simulink model "MSBR"  (R2015b)
settings: Solver=ode45  StartTime=0.0  StopTime=simtime  RelTol=1e-3
values from neighbouring files (symbols this model uses):
  a_b = 1.656E-05    (= 1.656e-05)    [Parameters_Core_PHE.m]    (also in Parameters_Core_PHE_FEHE.m; Parameters_MSBR.m)
  a_f = -8.172E-05    (= -8.172e-05)    [Parameters_Core_PHE.m]    (also in Parameters_Core_PHE_FEHE.m; Parameters_MSBR.m)
  a_g = 2.016E-05    (= 2.016e-05)    [Parameters_Core_PHE.m]    (also in Parameters_Core_PHE_FEHE.m; Parameters_MSBR.m)
  beta = [2.290E-04, 8.320E-04, 7.100E-04, 8.520E-04, 1.710E-04, 1.020E-04]    [Parameters_Core_PHE.m]    (also in Parameters_Core_PHE_FEHE.m; Parameters_MSBR.m)
  beta_t = sum(beta)    [Parameters_Core_PHE.m]    (also in Parameters_Core_PHE_FEHE.m; Parameters_MSBR.m)
  hA_bg = 1.054E+00    (= 1.054)    [Parameters_Core_PHE.m]    (also in Parameters_Core_PHE_FEHE.m; Parameters_MSBR.m)
  hA_fg_dn = 1.123E+00    (= 1.123)    [Parameters_Core_PHE.m]    (also in Parameters_Core_PHE_FEHE.m; Parameters_MSBR.m)
  hA_fg_up = 1.733E+00    (= 1.733)    [Parameters_Core_PHE.m]    (also in Parameters_Core_PHE_FEHE.m; Parameters_MSBR.m)
  hA_p1 = 0.75*3.030    (= 2.2725)    [Parameters_Core_PHE.m]    (also in Parameters_Core_PHE_FEHE.m = 2.993352; Parameters_MSBR.m = 2.993352; Parameters_PHE.m = 3.03)
  hA_p2 = 0.75*3.030    (= 2.2725)    [Parameters_Core_PHE.m]    (also in Parameters_Core_PHE_FEHE.m = 2.993352; Parameters_MSBR.m = 2.993352; Parameters_PHE.m = 3.03)
  hA_p3 = 0.75*3.030    (= 2.2725)    [Parameters_Core_PHE.m]    (also in Parameters_Core_PHE_FEHE.m = 2.993352; Parameters_MSBR.m = 2.993352; Parameters_PHE.m = 3.03)
  hA_p4 = 0.75*3.030    (= 2.2725)    [Parameters_Core_PHE.m]    (also in Parameters_Core_PHE_FEHE.m = 2.993352; Parameters_MSBR.m = 2.993352; Parameters_PHE.m = 3.03)
  hA_pb1 = 7.150E-01    (= 0.715)    [Parameters_Core_PHE_FEHE.m]    (also in Parameters_MSBR.m)
  hA_pb2 = 7.150E-01    (= 0.715)    [Parameters_Core_PHE_FEHE.m]    (also in Parameters_MSBR.m)
  hA_s1 = 0.75*5.929    (= 4.44675)    [Parameters_Core_PHE.m]    (also in Parameters_Core_PHE_FEHE.m = 5.85606; Parameters_MSBR.m = 5.85606; Parameters_PHE.m = 5.929)
  hA_s2 = 0.75*5.929    (= 4.44675)    [Parameters_Core_PHE.m]    (also in Parameters_Core_PHE_FEHE.m = 5.85606; Parameters_MSBR.m = 5.85606; Parameters_PHE.m = 5.929)
  hA_s3 = 0.75*5.929    (= 4.44675)    [Parameters_Core_PHE.m]    (also in Parameters_Core_PHE_FEHE.m = 5.85606; Parameters_MSBR.m = 5.85606; Parameters_PHE.m = 5.929)
  hA_s4 = 0.75*5.929    (= 4.44675)    [Parameters_Core_PHE.m]    (also in Parameters_Core_PHE_FEHE.m = 5.85606; Parameters_MSBR.m = 5.85606; Parameters_PHE.m = 5.929)
  hA_s5 = 7.150E-01    (= 0.715)    [Parameters_Core_PHE_FEHE.m]    (also in Parameters_MSBR.m)
  hA_s6 = 7.150E-01    (= 0.715)    [Parameters_Core_PHE_FEHE.m]    (also in Parameters_MSBR.m)
  k_1 = 5.000E-01    (= 0.5)    [Parameters_Core_PHE.m]    (also in Parameters_Core_PHE_FEHE.m; Parameters_MSBR.m)
  k_1b = 5.000E-01    (= 0.5)    [Parameters_Core_PHE.m]    (also in Parameters_Core_PHE_FEHE.m; Parameters_MSBR.m)
  k_2 = 5.000E-01    (= 0.5)    [Parameters_Core_PHE.m]    (also in Parameters_Core_PHE_FEHE.m; Parameters_MSBR.m)
  k_2b = 5.000E-01    (= 0.5)    [Parameters_Core_PHE.m]    (also in Parameters_Core_PHE_FEHE.m; Parameters_MSBR.m)
  k_3 = 5.000E-01    (= 0.5)    [Parameters_Core_PHE.m]    (also in Parameters_Core_PHE_FEHE.m; Parameters_MSBR.m)
  k_4 = 5.000E-01    (= 0.5)    [Parameters_Core_PHE.m]    (also in Parameters_Core_PHE_FEHE.m; Parameters_MSBR.m)
  k_b1 = 8.500E-03    (= 0.0085)    [Parameters_Core_PHE.m]    (also in Parameters_Core_PHE_FEHE.m; Parameters_MSBR.m)
  k_b2 = 8.500E-03    (= 0.0085)    [Parameters_Core_PHE.m]    (also in Parameters_Core_PHE_FEHE.m; Parameters_MSBR.m)
  k_f1 = 2.210E-01    (= 0.221)    [Parameters_Core_PHE.m]    (also in Parameters_Core_PHE_FEHE.m; Parameters_MSBR.m)
  k_f2 = 2.210E-01    (= 0.221)    [Parameters_Core_PHE.m]    (also in Parameters_Core_PHE_FEHE.m; Parameters_MSBR.m)
  k_f3 = 2.210E-01    (= 0.221)    [Parameters_Core_PHE.m]    (also in Parameters_Core_PHE_FEHE.m; Parameters_MSBR.m)
  k_f4 = 2.210E-01    (= 0.221)    [Parameters_Core_PHE.m]    (also in Parameters_Core_PHE_FEHE.m; Parameters_MSBR.m)
  k_g1 = 3.300E-02    (= 0.033)    [Parameters_Core_PHE.m]    (also in Parameters_Core_PHE_FEHE.m; Parameters_MSBR.m)
  k_g2 = 3.300E-02    (= 0.033)    [Parameters_Core_PHE.m]    (also in Parameters_Core_PHE_FEHE.m; Parameters_MSBR.m)
  k_g3 = 8.140E-03    (= 0.00814)    [Parameters_Core_PHE.m]    (also in Parameters_Core_PHE_FEHE.m; Parameters_MSBR.m)
  Lam = 3.300E-04    (= 0.00033)    [Parameters_Core_PHE.m]    (also in Parameters_Core_PHE_FEHE.m; Parameters_MSBR.m)
  lam = [1.260E-02, 3.370E-02, 1.390E-01, 3.250E-01, 1.130E+00, 2.500E+00]    [Parameters_Core_PHE.m]    (also in Parameters_Core_PHE_FEHE.m; Parameters_MSBR.m)
  mb_cpb = 3.297E+01    (= 32.97)    [Parameters_Core_PHE_FEHE.m]    (also in Parameters_MSBR.m)
  mcp_b1 = 1.733E+00    (= 1.733)    [Parameters_Core_PHE.m]    (also in Parameters_Core_PHE_FEHE.m; Parameters_MSBR.m)
  mcp_b2 = 1.733E+00    (= 1.733)    [Parameters_Core_PHE.m]    (also in Parameters_Core_PHE_FEHE.m; Parameters_MSBR.m)
  mcp_f1 = 2.748E-01    (= 0.2748)    [Parameters_Core_PHE.m]    (also in Parameters_Core_PHE_FEHE.m; Parameters_MSBR.m)
  mcp_f2 = 2.748E-01    (= 0.2748)    [Parameters_Core_PHE.m]    (also in Parameters_Core_PHE_FEHE.m; Parameters_MSBR.m)
  mcp_f3 = 2.748E-01    (= 0.2748)    [Parameters_Core_PHE.m]    (also in Parameters_Core_PHE_FEHE.m; Parameters_MSBR.m)
  mcp_f4 = 2.748E-01    (= 0.2748)    [Parameters_Core_PHE.m]    (also in Parameters_Core_PHE_FEHE.m; Parameters_MSBR.m)
  mcp_g1 = 1.403E+01    (= 14.03)    [Parameters_Core_PHE.m]    (also in Parameters_Core_PHE_FEHE.m; Parameters_MSBR.m)
  mcp_g2 = 1.403E+01    (= 14.03)    [Parameters_Core_PHE.m]    (also in Parameters_Core_PHE_FEHE.m; Parameters_MSBR.m)
  mcp_g3 = 3.467E+00    (= 3.467)    [Parameters_Core_PHE.m]    (also in Parameters_Core_PHE_FEHE.m; Parameters_MSBR.m)
  mcp_p1 = mn_p*cp_p    (= 1.743765)    [Parameters_Core_PHE.m]    (also in Parameters_Core_PHE_FEHE.m; Parameters_MSBR.m; Parameters_PHE.m = 0.930008)
  mcp_p2 = mn_p*cp_p    (= 1.743765)    [Parameters_Core_PHE.m]    (also in Parameters_Core_PHE_FEHE.m; Parameters_MSBR.m; Parameters_PHE.m = 0.930008)
  mcp_p3 = mn_p*cp_p    (= 1.743765)    [Parameters_Core_PHE.m]    (also in Parameters_Core_PHE_FEHE.m; Parameters_MSBR.m; Parameters_PHE.m = 0.930008)
  mcp_p4 = mn_p*cp_p    (= 1.743765)    [Parameters_Core_PHE.m]    (also in Parameters_Core_PHE_FEHE.m; Parameters_MSBR.m; Parameters_PHE.m = 0.930008)
  mcp_pb1 = 3.967E-01    (= 0.3967)    [Parameters_Core_PHE_FEHE.m]    (also in Parameters_MSBR.m)
  mcp_pb2 = 3.967E-01    (= 0.3967)    [Parameters_Core_PHE_FEHE.m]    (also in Parameters_MSBR.m)
  mcp_s1 = mn_s*cp_s    (= 6.80458)    [Parameters_Core_PHE.m]    (also in Parameters_Core_PHE_FEHE.m; Parameters_MSBR.m; Parameters_PHE.m)
  mcp_s2 = mn_s*cp_s    (= 6.80458)    [Parameters_Core_PHE.m]    (also in Parameters_Core_PHE_FEHE.m; Parameters_MSBR.m; Parameters_PHE.m)
  mcp_s3 = mn_s*cp_s    (= 6.80458)    [Parameters_Core_PHE.m]    (also in Parameters_Core_PHE_FEHE.m; Parameters_MSBR.m; Parameters_PHE.m)
  mcp_s4 = mn_s*cp_s    (= 6.80458)    [Parameters_Core_PHE.m]    (also in Parameters_Core_PHE_FEHE.m; Parameters_MSBR.m; Parameters_PHE.m)
  mcp_s5 = 2.632E+00    (= 2.632)    [Parameters_Core_PHE_FEHE.m]    (also in Parameters_MSBR.m)
  mcp_s6 = 2.632E+00    (= 2.632)    [Parameters_Core_PHE_FEHE.m]    (also in Parameters_MSBR.m)
  mcp_t1 = 2.158    [Parameters_Core_PHE.m]    (also in Parameters_Core_PHE_FEHE.m; Parameters_MSBR.m; Parameters_PHE.m)
  mcp_t2 = 2.158    [Parameters_Core_PHE.m]    (also in Parameters_Core_PHE_FEHE.m; Parameters_MSBR.m; Parameters_PHE.m)
  mcp_t3 = m_t*cp_t    (= 0.51412242)    [Parameters_Core_PHE_FEHE.m]    (also in Parameters_MSBR.m)
  mn_m = 1.414e3    (= 1414)    [Parameters_Core_PHE.m]    (also in Parameters_Core_PHE_FEHE.m; Parameters_MSBR.m; Parameters_PHE.m)
  mn_ms = mn_m    (= 1414)    [Parameters_Core_PHE_FEHE.m]    (also in Parameters_MSBR.m)
  mn_p = m_p/nn_p    (= 757.5)    [Parameters_Core_PHE.m]    (also in Parameters_Core_PHE_FEHE.m; Parameters_MSBR.m; Parameters_PHE.m = 404)
  mn_s = m_s/nn_s    (= 3970)    [Parameters_Core_PHE.m]    (also in Parameters_Core_PHE_FEHE.m; Parameters_MSBR.m; Parameters_PHE.m)
  mr_cpr = 1.050E+01    (= 10.5)    [Parameters_Core_PHE_FEHE.m]    (also in Parameters_MSBR.m)
  n_frac0 = 1    [Parameters_Core_PHE.m]    (also in Parameters_Core_PHE_FEHE.m; Parameters_MSBR.m)
  P = 556.0    (= 556)    [Parameters_Core_PHE.m]    (also in Parameters_Core_PHE_FEHE.m; Parameters_MSBR.m)
  p_b = 0.87*P    (= 483.72)    [Parameters_Core_PHE_FEHE.m]    (also in Parameters_MSBR.m)
  p_r = 0.13*P    (= 72.28)    [Parameters_Core_PHE_FEHE.m]    (also in Parameters_MSBR.m)
  T0_b1 = 648.88    [Parameters_Core_PHE.m]    (also in Parameters_Core_PHE_FEHE.m; Parameters_MSBR.m)
  T0_b2 = 676.66    [Parameters_Core_PHE.m]    (also in Parameters_Core_PHE_FEHE.m; Parameters_MSBR.m)
  T0_f1 = 579.44    [Parameters_Core_PHE.m]    (also in Parameters_Core_PHE_FEHE.m; Parameters_MSBR.m)
  T0_f2 = 621.11    [Parameters_Core_PHE.m]    (also in Parameters_Core_PHE_FEHE.m; Parameters_MSBR.m)
  T0_f3 = 662.77    [Parameters_Core_PHE.m]    (also in Parameters_Core_PHE_FEHE.m; Parameters_MSBR.m)
  T0_f4 = 704.44    [Parameters_Core_PHE.m]    (also in Parameters_Core_PHE_FEHE.m; Parameters_MSBR.m)
  T0_g1 = 590.00    (= 590)    [Parameters_Core_PHE.m]    (also in Parameters_Core_PHE_FEHE.m; Parameters_MSBR.m)
  T0_g2 = 673.33    [Parameters_Core_PHE.m]    (also in Parameters_Core_PHE_FEHE.m; Parameters_MSBR.m)
  T0_g3 = 652.77    [Parameters_Core_PHE.m]    (also in Parameters_Core_PHE_FEHE.m; Parameters_MSBR.m)
  T0_p1 = Tp_in - 41.6675    (= 662.7725)    [Parameters_Core_PHE.m]    (also in Parameters_Core_PHE_FEHE.m; Parameters_MSBR.m; Parameters_PHE.m)
  T0_p2 = Tp_in - 2*41.6675    (= 621.105)    [Parameters_Core_PHE.m]    (also in Parameters_Core_PHE_FEHE.m; Parameters_MSBR.m; Parameters_PHE.m)
  T0_p3 = Tp_in - 3*41.6675    (= 579.4375)    [Parameters_Core_PHE.m]    (also in Parameters_Core_PHE_FEHE.m; Parameters_MSBR.m; Parameters_PHE.m)
  T0_p4 = 537.77    [Parameters_Core_PHE.m]    (also in Parameters_Core_PHE_FEHE.m; Parameters_MSBR.m; Parameters_PHE.m)
  T0_pb1 = 648.88    [Parameters_Core_PHE_FEHE.m]    (also in Parameters_MSBR.m)
  T0_pb2 = 676.66    [Parameters_Core_PHE_FEHE.m]    (also in Parameters_MSBR.m)
  T0_pm = T0_p2    (= 621.105)    [Parameters_Core_PHE.m]    (also in Parameters_Core_PHE_FEHE.m; Parameters_MSBR.m; Parameters_PHE.m)
  T0_s1 = Ts_in + 36.25    (= 490.694)    [Parameters_Core_PHE.m]    (also in Parameters_Core_PHE_FEHE.m; Parameters_MSBR.m; Parameters_PHE.m)
  T0_s2 = Ts_in + 2*36.25    (= 526.944)    [Parameters_Core_PHE.m]    (also in Parameters_Core_PHE_FEHE.m; Parameters_MSBR.m; Parameters_PHE.m)
  T0_s3 = Ts_in + 3*36.25    (= 563.194)    [Parameters_Core_PHE.m]    (also in Parameters_Core_PHE_FEHE.m; Parameters_MSBR.m; Parameters_PHE.m)
  T0_s4 = 599.4444    [Parameters_Core_PHE.m]    (also in Parameters_Core_PHE_FEHE.m; Parameters_MSBR.m; Parameters_PHE.m)
  T0_s5 = 603.33    [Parameters_Core_PHE_FEHE.m]    (also in Parameters_MSBR.m)
  T0_s6 = 607.22    [Parameters_Core_PHE_FEHE.m]    (also in Parameters_MSBR.m)
  T0_t1 = 596.87    [Parameters_Core_PHE.m]    (also in Parameters_Core_PHE_FEHE.m; Parameters_MSBR.m; Parameters_PHE.m)
  T0_t2 = 520.71    [Parameters_Core_PHE.m]    (also in Parameters_Core_PHE_FEHE.m; Parameters_MSBR.m; Parameters_PHE.m)
  T0_t3 = 633.6967    [Parameters_Core_PHE_FEHE.m]    (also in Parameters_MSBR.m)
  tau_1 = mn_f/W_f    (= 0.084441301273)    [Parameters_Core_PHE.m]    (also in Parameters_Core_PHE_FEHE.m; Parameters_MSBR.m)
  tau_2 = mn_f/W_f    (= 0.084441301273)    [Parameters_Core_PHE.m]    (also in Parameters_Core_PHE_FEHE.m; Parameters_MSBR.m)
  tau_3 = mn_f/W_f    (= 0.084441301273)    [Parameters_Core_PHE.m]    (also in Parameters_Core_PHE_FEHE.m; Parameters_MSBR.m)
  tau_4 = mn_f/W_f    (= 0.084441301273)    [Parameters_Core_PHE.m]    (also in Parameters_Core_PHE_FEHE.m; Parameters_MSBR.m)
  tau_b = 10.43    [Parameters_Core_PHE_FEHE.m]    (also in Parameters_MSBR.m)
  tau_b1 = 6.998E+00    (= 6.998)    [Parameters_Core_PHE.m]    (also in Parameters_Core_PHE_FEHE.m; Parameters_MSBR.m)
  tau_b2 = 6.998E+00    (= 6.998)    [Parameters_Core_PHE.m]    (also in Parameters_Core_PHE_FEHE.m; Parameters_MSBR.m)
  tau_b_fhx = 4.2    [Parameters_Core_PHE.m]    (also in Parameters_Core_PHE_FEHE.m; Parameters_MSBR.m)
  tau_c = 3.28    [Parameters_Core_PHE.m]    (also in Parameters_Core_PHE_FEHE.m; Parameters_MSBR.m)
  tau_c_fehx = 7.0    (= 7)    [Parameters_Core_PHE.m]    (also in Parameters_Core_PHE_FEHE.m; Parameters_MSBR.m)
  tau_c_fhx = 1.32    [Parameters_Core_PHE.m]    (also in Parameters_Core_PHE_FEHE.m; Parameters_MSBR.m)
  tau_fehx_b = 13.5    [Parameters_Core_PHE.m]    (also in Parameters_Core_PHE_FEHE.m; Parameters_MSBR.m)
  tau_fehx_c = 7.0    (= 7)    [Parameters_Core_PHE.m]    (also in Parameters_Core_PHE_FEHE.m; Parameters_MSBR.m)
  tau_fehx_r = 17.3    [Parameters_Core_PHE.m]    (also in Parameters_Core_PHE_FEHE.m; Parameters_MSBR.m)
  tau_fhx_c = 1.22    [Parameters_Core_PHE.m]    (also in Parameters_Core_PHE_FEHE.m; Parameters_MSBR.m)
  tau_fhx_fehx = 7.88    [Parameters_Core_PHE.m]    (also in Parameters_Core_PHE_FEHE.m; Parameters_MSBR.m)
  tau_l = 5.85    [Parameters_Core_PHE.m]    (also in Parameters_Core_PHE_FEHE.m; Parameters_MSBR.m)
  tau_pb = 7.983E-01    (= 0.7983)    [Parameters_Core_PHE_FEHE.m]    (also in Parameters_MSBR.m)
  tau_r = 22.09    [Parameters_Core_PHE_FEHE.m]    (also in Parameters_MSBR.m)
  tau_r_fhx = 11.1    [Parameters_Core_PHE.m]    (also in Parameters_Core_PHE_FEHE.m; Parameters_MSBR.m)
  tau_s5 = 7.446E-01    (= 0.7446)    [Parameters_Core_PHE_FEHE.m]    (also in Parameters_MSBR.m)
  tau_s6 = 7.446E-01    (= 0.7446)    [Parameters_Core_PHE_FEHE.m]    (also in Parameters_MSBR.m)
  Ts_in = 454.444    [Parameters_Core_PHE.m]    (also in Parameters_Core_PHE_FEHE.m; Parameters_MSBR.m; Parameters_PHE.m)
  W_p = 1.414E3    (= 1414)    [Parameters_Core_PHE.m]    (also in Parameters_Core_PHE_FEHE.m; Parameters_MSBR.m; Parameters_PHE.m)
  ... (+3 more)
undefined symbols (not defined in the file or in its folder): C0
libraries: simulink x2
settings Model: Creator=mlish  LastModifiedBy=mlish
settings DataIOCC: LimitDataPoints=off

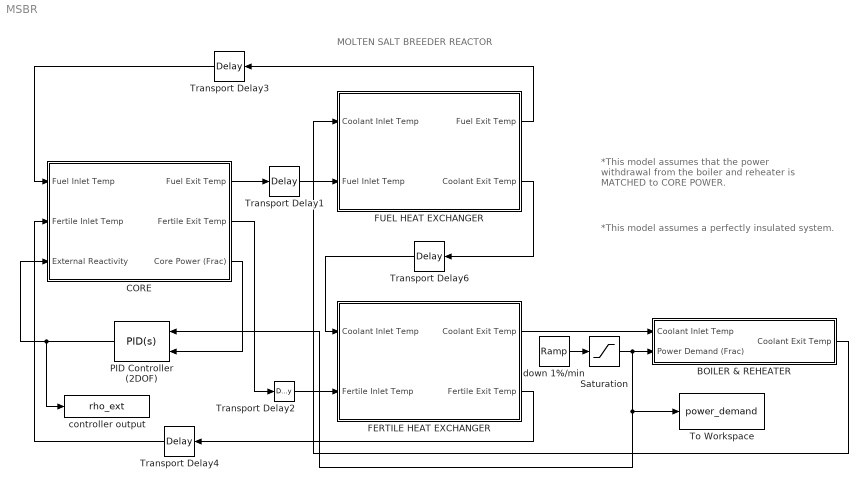
== system MSBR ==
  note: *This model assumes a perfectly insulated system.
  note: MOLTEN SALT BREEDER REACTOR
  note: *This model assumes that the power
      | withdrawal from the boiler and reheater
      | is MATCHED to CORE POWER.
  BOILER & REHEATER : Subsystem
  CORE : Subsystem
  FERTILE HEAT EXCHANGER : Subsystem
  FUEL HEAT EXCHANGER : Subsystem
  PID Controller (2DOF) : simulink/Continuous/PID Controller (2DOF)  Controller=PID  TimeDomain=Continuous-time  SampleTime=-1  IntegratorMethod=Forward Euler  FilterMethod=Forward Euler  Form=Parallel  UseFilter=on  ControllerParametersSource=internal  P=0  I=0.00870790380431012  D=0  N=100  b=1  c=1  InitialConditionSource=internal  InitialConditionForIntegrator=0  InitialConditionForFilter=0  ExternalReset=none  LimitOutput=off  UpperSaturationLimit=inf  LowerSaturationLimit=-inf  LinearizeAsGain=on  AntiWindupMode=none  Kb=1  TrackingMode=off  Kt=1  PParamMin=[]  PParamMax=[]  IParamMin=[]  IParamMax=[]  DParamMin=[]  DParamMax=[]  NParamMin=[]  NParamMax=[]  bParamMin=[]  bParamMax=[]  cParamMin=[]  cParamMax=[]  KbParamMin=[]  KbParamMax=[]  KtParamMin=[]  KtParamMax=[]  POutMin=[]  POutMax=[]  IOutMin=[]  IOutMax=[]  DOutMin=[]  DOutMax=[]  NOutMin=[]  NOutMax=[]  bOutMin=[]  bOutMax=[]  cOutMin=[]  cOutMax=[]  KbOutMin=[]  KbOutMax=[]  KtOutMin=[]  KtOutMax=[]  IntegratorOutMin=[]  IntegratorOutMax=[]  FilterOutMin=[]  FilterOutMax=[]  SumOutMin=[]  SumOutMax=[]  Sum1OutMin=[]  Sum1OutMax=[]  Sum2OutMin=[]  Sum2OutMax=[]  Sum3OutMin=[]  Sum3OutMax=[]  SumI1OutMin=[]  SumI1OutMax=[]  SumI2OutMin=[]  SumI2OutMax=[]  SumI3OutMin=[]  SumI3OutMax=[]  SumDOutMin=[]  SumDOutMax=[]  SaturationOutMin=[]  SaturationOutMax=[]  IntegratorContinuousStateAttributes=''  IntegratorStateMustResolveToSignalObject=off  IntegratorRTWStateStorageClass=Auto  FilterContinuousStateAttributes=''  FilterStateMustResolveToSignalObject=off  FilterRTWStateStorageClass=Auto  DifferentiatorICPrevScaledInput=0  DifferentiatorOutMin=[]  DifferentiatorOutMax=[]
  Saturation : Saturate  UpperLimit=1  LowerLimit=0.9
  To Workspace : ToWorkspace  VariableName=power_demand  SampleTime=-1
  Transport Delay1 : TransportDelay  DelayTime=tau_c_fhx  InitialOutput=T0_f4  BufferSize=4096
  Transport Delay2 : TransportDelay  DelayTime=tau_c_fehx  InitialOutput=T0_b2  BufferSize=4096
  Transport Delay3 : TransportDelay  DelayTime=tau_fhx_c  InitialOutput=T0_p4  BufferSize=4096
  Transport Delay4 : TransportDelay  DelayTime=tau_fehx_c  InitialOutput=T0_pb2  BufferSize=4096
  Transport Delay6 : TransportDelay  DelayTime=tau_fhx_fehx  InitialOutput=T0_s4  BufferSize=4096
  controller output : ToWorkspace  VariableName=rho_ext  SampleTime=-1
  down 1%/min : simulink/Sources/Ramp  slope=-0.01/60  start=400  X0=1
  wires:
  FUEL HEAT EXCHANGER/2(Coolant Exit Temp) -> Transport Delay6/1
  FERTILE HEAT EXCHANGER/2(Fertile Exit Temp) -> Transport Delay4/1
  FERTILE HEAT EXCHANGER/1(Coolant Exit Temp) -> BOILER & REHEATER/1(Coolant Inlet Temp)
  Transport Delay1/1 -> FUEL HEAT EXCHANGER/2(Fuel Inlet Temp)
  CORE/1(Fuel Exit Temp) -> Transport Delay1/1
  CORE/2(Fertile Exit Temp) -> Transport Delay2/1
  Transport Delay2/1 -> FERTILE HEAT EXCHANGER/2(Fertile Inlet Temp)
  Transport Delay3/1 -> CORE/1(Fuel Inlet Temp)
  FUEL HEAT EXCHANGER/1(Fuel Exit Temp) -> Transport Delay3/1
  Transport Delay6/1 -> FERTILE HEAT EXCHANGER/1(Coolant Inlet Temp)
  Transport Delay4/1 -> CORE/2(Fertile Inlet Temp)
  BOILER & REHEATER/1(Coolant Exit Temp) -> FUEL HEAT EXCHANGER/1(Coolant Inlet Temp)
  Saturation/1 -> PID Controller (2DOF)/1, To Workspace/1, BOILER & REHEATER/2(Power Demand (Frac))
  down 1%/min/1 -> Saturation/1
  CORE/3(Core Power (Frac)) -> PID Controller (2DOF)/2
  PID Controller (2DOF)/1 -> controller output/1, CORE/3(External Reactivity)

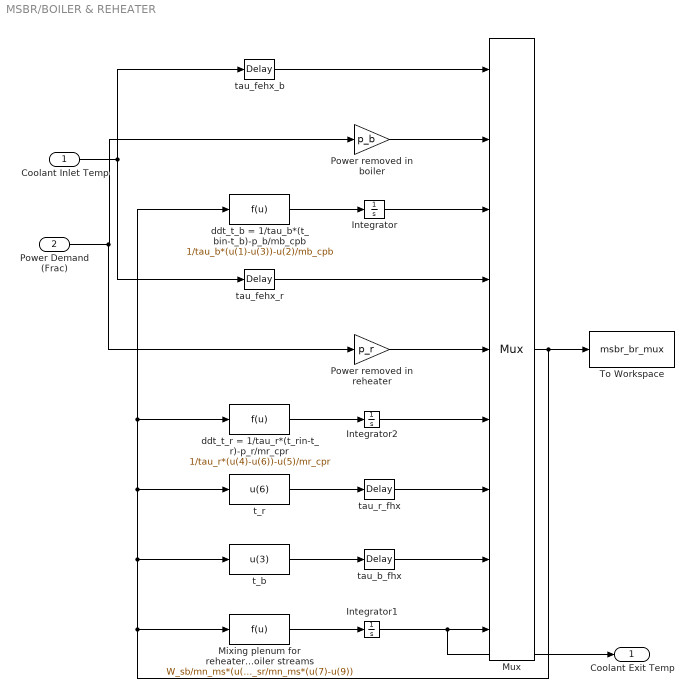
== system MSBR/BOILER & REHEATER ==
  Coolant Inlet Temp : Inport
  Power Demand (Frac) : Inport  Port=2
  Integrator : Integrator  InitialCondition=Ts_in
  Integrator1 : Integrator  InitialCondition=Ts_in
  Integrator2 : Integrator  InitialCondition=Ts_in
  Mixing plenum for reheater and boiler streams : Fcn  Expr=W_sb/mn_ms*(u(8)-u(9))+W_sr/mn_ms*(u(7)-u(9))
  Mux : Mux  Inputs=9
      settings: DisplayOption=signals
  Power removed in boiler : Gain  Gain=p_b
  Power removed in reheater : Gain  Gain=p_r
  To Workspace : ToWorkspace  VariableName=msbr_br_mux  SampleTime=-1
  ddt_t_b = 1/tau_b*(t_bin-t_b)-p_b/mb_cpb : Fcn  Expr=1/tau_b*(u(1)-u(3))-u(2)/mb_cpb
  ddt_t_r = 1/tau_r*(t_rin-t_r)-p_r/mr_cpr : Fcn  Expr=1/tau_r*(u(4)-u(6))-u(5)/mr_cpr
  t_b : Fcn  Expr=u(3)
  t_r : Fcn  Expr=u(6)
  tau_b_fhx : TransportDelay  DelayTime=tau_b_fhx  InitialOutput=Ts_in  BufferSize=4096
  tau_fehx_b : TransportDelay  DelayTime=tau_fehx_b  InitialOutput=T0_s6  BufferSize=4096
  tau_fehx_r : TransportDelay  DelayTime=tau_fehx_r  InitialOutput=T0_s6  BufferSize=4096
  tau_r_fhx : TransportDelay  DelayTime=tau_r_fhx  InitialOutput=Ts_in  BufferSize=4096
  Coolant Exit Temp : Outport
  wires:
  Coolant Inlet Temp/1 -> tau_fehx_r/1, tau_fehx_b/1
  Power removed in boiler/1 -> Mux/2
  Integrator/1 -> Mux/3
  ddt_t_r = 1/tau_r*(t_rin-t_r)-p_r/mr_cpr/1 -> Integrator2/1
  ddt_t_b = 1/tau_b*(t_bin-t_b)-p_b/mb_cpb/1 -> Integrator/1
  Mux/1 -> t_b/1, t_r/1, ddt_t_r = 1/tau_r*(t_rin-t_r)-p_r/mr_cpr/1, ddt_t_b = 1/tau_b*(t_bin-t_b)-p_b/mb_cpb/1, Mixing plenum for reheater and boiler streams/1, To Workspace/1
  tau_fehx_r/1 -> Mux/4
  Power removed in reheater/1 -> Mux/5
  Integrator2/1 -> Mux/6
  Mixing plenum for reheater and boiler streams/1 -> Integrator1/1
  Integrator1/1 -> Coolant Exit Temp/1, Mux/9
  tau_b_fhx/1 -> Mux/8
  tau_r_fhx/1 -> Mux/7
  t_r/1 -> tau_r_fhx/1
  t_b/1 -> tau_b_fhx/1
  tau_fehx_b/1 -> Mux/1
  Power Demand (Frac)/1 -> Power removed in reheater/1, Power removed in boiler/1

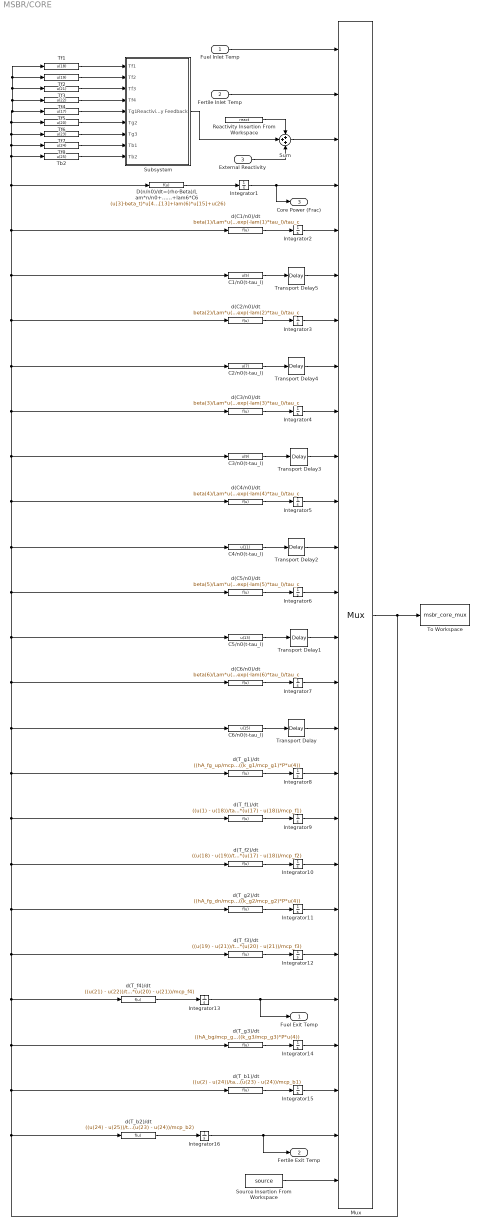
== system MSBR/CORE ==
  Fuel Inlet Temp : Inport
  Fertile Inlet Temp : Inport  Port=2
  External Reactivity : Inport  Port=3
  C1/n0(t-tau_l) : Fcn  Expr=u(5)
  C2/n0(t-tau_l) : Fcn  Expr=u(7)
  C3/n0(t-tau_l) : Fcn  Expr=u(9)
  C4/n0(t-tau_l) : Fcn  Expr=u(11)
  C5/n0(t-tau_l) : Fcn  Expr=u(13)
  C6/n0(t-tau_l) : Fcn  Expr=u(15)
  D(n/n0)/dt=(rho-Beta)/Lam*n/n0+lam1*C1+...+lam6*C6 : Fcn  Expr=(u[3]-beta_t)*u[4]/Lam+lam(1)*u[5]+lam(2)*u[7]+lam(3)*u[9]+lam(4)*u[11]+lam(5)*u[13]+lam(6)*u[15]+u(26)
  Integrator1 : Integrator  InitialCondition=n_frac0
  Integrator10 : Integrator  InitialCondition=T0_f2
  Integrator11 : Integrator  InitialCondition=T0_g2
  Integrator12 : Integrator  InitialCondition=T0_f3
  Integrator13 : Integrator  InitialCondition=T0_f4
  Integrator14 : Integrator  InitialCondition=T0_g3
  Integrator15 : Integrator  InitialCondition=T0_b1
  Integrator16 : Integrator  InitialCondition=T0_b2
  Integrator2 : Integrator  InitialCondition=C0(1)
  Integrator3 : Integrator  InitialCondition=C0(2)
  Integrator4 : Integrator  InitialCondition=C0(3)
  Integrator5 : Integrator  InitialCondition=C0(4)
  Integrator6 : Integrator  InitialCondition=C0(5)
  Integrator7 : Integrator  InitialCondition=C0(6)
  Integrator8 : Integrator  InitialCondition=T0_g1
  Integrator9 : Integrator  InitialCondition=T0_f1
  Mux : Mux  Inputs=26
      settings: DisplayOption=signals
  Reactivity Insertion From Workspace : FromWorkspace  VariableName=react  SampleTime=1  Interpolate=off  OutputAfterFinalValue=Holding final value
  Source Insertion From Workspace : FromWorkspace  VariableName=source  SampleTime=1  Interpolate=off  OutputAfterFinalValue=Holding final value
  Subsystem : Subsystem
  Sum : Sum  Inputs=+++
  Tb2 : Fcn  Expr=u(25)
  Tf1 : Fcn  Expr=u(18)
  Tf2 : Fcn  Expr=u(19)
  Tf3 : Fcn  Expr=u(21)
  Tf4 : Fcn  Expr=u(22)
  Tf5 : Fcn  Expr=u(17)
  Tf6 : Fcn  Expr=u(20)
  Tf7 : Fcn  Expr=u(23)
  Tf8 : Fcn  Expr=u(24)
  To Workspace : ToWorkspace  VariableName=msbr_core_mux  SampleTime=-1
  Transport Delay : TransportDelay  DelayTime=tau_l  InitialOutput=C0(6)  BufferSize=4096
  Transport Delay1 : TransportDelay  DelayTime=tau_l  InitialOutput=C0(5)  BufferSize=4096
  Transport Delay2 : TransportDelay  DelayTime=tau_l  InitialOutput=C0(4)  BufferSize=4096
  Transport Delay3 : TransportDelay  DelayTime=tau_l  InitialOutput=C0(3)  BufferSize=4096
  Transport Delay4 : TransportDelay  DelayTime=tau_l  InitialOutput=C0(2)  BufferSize=4096
  Transport Delay5 : TransportDelay  DelayTime=tau_l  InitialOutput=C0(1)  BufferSize=4096
  d(C1/n0)/dt : Fcn  Expr=beta(1)/Lam*u(4)-lam(1)*u(5)-u(5)/tau_c+u(6)*exp(-lam(1)*tau_l)/tau_c
  d(C2/n0)/dt : Fcn  Expr=beta(2)/Lam*u(4)-lam(2)*u(7)-u(7)/tau_c+u(8)*exp(-lam(2)*tau_l)/tau_c
  d(C3/n0)/dt : Fcn  Expr=beta(3)/Lam*u(4)-lam(3)*u(9)-u(9)/tau_c+u(10)*exp(-lam(3)*tau_l)/tau_c
  d(C4/n0)/dt : Fcn  Expr=beta(4)/Lam*u(4)-lam(4)*u(11)-u(11)/tau_c+u(12)*exp(-lam(4)*tau_l)/tau_c
  d(C5/n0)/dt : Fcn  Expr=beta(5)/Lam*u(4)-lam(5)*u(13)-u(13)/tau_c+u(14)*exp(-lam(5)*tau_l)/tau_c
  d(C6/n0)/dt : Fcn  Expr=beta(6)/Lam*u(4)-lam(6)*u(15)-u(15)/tau_c+u(16)*exp(-lam(6)*tau_l)/tau_c
  d(T_b1)/dt : Fcn  Expr=((u(2) - u(24))/tau_b1) + (k_b1*P*u(4)/mcp_b1) + (hA_bg*k_1b*(u(23) - u(24))/mcp_b1)
  d(T_b2)/dt : Fcn  Expr=((u(24) - u(25))/tau_b2) + (k_b2*P*u(4)/mcp_b2) + (hA_bg*k_2b*(u(23) - u(24))/mcp_b2)
  d(T_f1)/dt : Fcn  Expr=((u(1) - u(18))/tau_1) + (k_f1*P*u(4)/mcp_f1) + (hA_fg_up*k_1*(u(17) - u(18))/mcp_f1)
  d(T_f2)/dt : Fcn  Expr=((u(18) - u(19))/tau_2) + (k_f2*P*u(4)/mcp_f2) + (hA_fg_up*k_2*(u(17) - u(18))/mcp_f2)
  d(T_f3)/dt : Fcn  Expr="((u(19) - u(21))/tau_3) +  (k_f3*P*u(4)/mcp_f3) + (hA_fg_dn*k_3*(u(20) - u(21))/mcp_f3)"
  d(T_f4)/dt : Fcn  Expr="((u(21) - u(22))/tau_4) +  (k_f4*P*u(4)/mcp_f4) + (hA_fg_dn*k_4*(u(20) - u(21))/mcp_f4)"
  d(T_g1)/dt : Fcn  Expr=((hA_fg_up/mcp_g1)*(u(18) - u(17))) + ((k_g1/mcp_g1)*P*u(4))
  d(T_g2)/dt : Fcn  Expr=((hA_fg_dn/mcp_g2)*(u(21) - u(20))) + ((k_g2/mcp_g2)*P*u(4))
  d(T_g3)/dt : Fcn  Expr=((hA_bg/mcp_g3)*(u(24) - u(23))) + ((k_g3/mcp_g3)*P*u(4))
  Fuel Exit Temp : Outport
  Fertile Exit Temp : Outport  Port=2
  Core Power (Frac) : Outport  Port=3
  wires:
  Fuel Inlet Temp/1 -> Mux/1
  Fertile Inlet Temp/1 -> Mux/2
  d(T_g1)/dt/1 -> Integrator8/1
  d(T_f1)/dt/1 -> Integrator9/1
  d(T_f2)/dt/1 -> Integrator10/1
  d(T_g2)/dt/1 -> Integrator11/1
  d(T_f3)/dt/1 -> Integrator12/1
  d(T_f4)/dt/1 -> Integrator13/1
  d(T_g3)/dt/1 -> Integrator14/1
  d(T_b1)/dt/1 -> Integrator15/1
  d(T_b2)/dt/1 -> Integrator16/1
  Integrator16/1 -> Fertile Exit Temp/1, Mux/25
  Integrator15/1 -> Mux/24
  Integrator14/1 -> Mux/23
  Integrator13/1 -> Fuel Exit Temp/1, Mux/22
  Integrator12/1 -> Mux/21
  Integrator11/1 -> Mux/20
  Integrator10/1 -> Mux/19
  Integrator9/1 -> Mux/18
  Integrator8/1 -> Mux/17
  Source Insertion From Workspace/1 -> Mux/26
  D(n/n0)/dt=(rho-Beta)/Lam*n/n0+lam1*C1+...+lam6*C6/1 -> Integrator1/1
  d(C1/n0)/dt/1 -> Integrator2/1
  d(C2/n0)/dt/1 -> Integrator3/1
  d(C3/n0)/dt/1 -> Integrator4/1
  d(C4/n0)/dt/1 -> Integrator5/1
  d(C5/n0)/dt/1 -> Integrator6/1
  d(C6/n0)/dt/1 -> Integrator7/1
  Integrator1/1 -> Core Power (Frac)/1, Mux/4
  Integrator2/1 -> Mux/5
  Integrator3/1 -> Mux/7
  Integrator4/1 -> Mux/9
  Integrator5/1 -> Mux/11
  Integrator6/1 -> Mux/13
  Integrator7/1 -> Mux/15
  C6/n0(t-tau_l)/1 -> Transport Delay/1
  Transport Delay/1 -> Mux/16
  C5/n0(t-tau_l)/1 -> Transport Delay1/1
  Transport Delay1/1 -> Mux/14
  Transport Delay2/1 -> Mux/12
  C4/n0(t-tau_l)/1 -> Transport Delay2/1
  C3/n0(t-tau_l)/1 -> Transport Delay3/1
  Transport Delay3/1 -> Mux/10
  Transport Delay4/1 -> Mux/8
  C2/n0(t-tau_l)/1 -> Transport Delay4/1
  Transport Delay5/1 -> Mux/6
  C1/n0(t-tau_l)/1 -> Transport Delay5/1
  Sum/1 -> Mux/3
  Reactivity Insertion From Workspace/1 -> Sum/1
  External Reactivity/1 -> Sum/3
  Mux/1 -> d(T_b2)/dt/1, d(T_b1)/dt/1, d(T_g3)/dt/1, d(T_f4)/dt/1, d(T_f3)/dt/1, d(T_g2)/dt/1, d(T_f2)/dt/1, d(T_f1)/dt/1, d(T_g1)/dt/1, C6/n0(t-tau_l)/1, d(C6/n0)/dt/1, C5/n0(t-tau_l)/1, d(C5/n0)/dt/1, C4/n0(t-tau_l)/1, d(C4/n0)/dt/1, C3/n0(t-tau_l)/1, d(C3/n0)/dt/1, d(C2/n0)/dt/1, C1/n0(t-tau_l)/1, Tf1/1, Tf2/1, Tf3/1, Tf4/1, Tf5/1, Tf6/1, Tf7/1, Tf8/1, Tb2/1, D(n/n0)/dt=(rho-Beta)/Lam*n/n0+lam1*C1+...+lam6*C6/1, d(C1/n0)/dt/1, C2/n0(t-tau_l)/1, To Workspace/1
  Tf1/1 -> Subsystem/1(Tf1)
  Tf2/1 -> Subsystem/2(Tf2)
  Tf3/1 -> Subsystem/3(Tf3)
  Tb2/1 -> Subsystem/9(Tb2)
  Tf8/1 -> Subsystem/8(Tb1)
  Tf7/1 -> Subsystem/7(Tg3)
  Tf6/1 -> Subsystem/6(Tg2)
  Tf5/1 -> Subsystem/5(Tg1)
  Tf4/1 -> Subsystem/4(Tf4)
  Subsystem/1(Reactivity Feedback) -> Sum/2

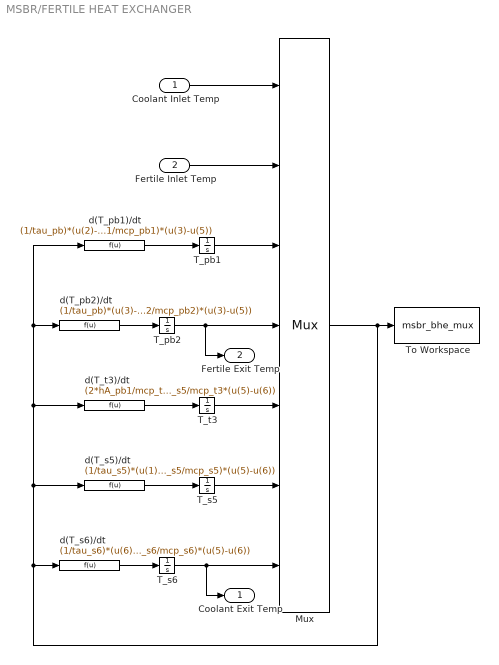
== system MSBR/FERTILE HEAT EXCHANGER ==
  Coolant Inlet Temp : Inport
  Fertile Inlet Temp : Inport  Port=2
  Mux : Mux  Inputs=7
      settings: DisplayOption=signals
  T_pb1 : Integrator  InitialCondition=T0_pb1
  T_pb2 : Integrator  InitialCondition=T0_pb2
  "T_s5 " : Integrator  InitialCondition=T0_s5
  T_s6 : Integrator  InitialCondition=T0_s6
  T_t3 : Integrator  InitialCondition=T0_t3
  To Workspace : ToWorkspace  VariableName=msbr_bhe_mux  SampleTime=-1
  d(T_pb1)/dt : Fcn  Expr=(1/tau_pb)*(u(2)-u(3))-(hA_pb1/mcp_pb1)*(u(3)-u(5))
  d(T_pb2)/dt : Fcn  Expr=(1/tau_pb)*(u(3)-u(4))-(hA_pb2/mcp_pb2)*(u(3)-u(5))
  d(T_s5)/dt : Fcn  Expr=(1/tau_s5)*(u(1)-u(6))+(hA_s5/mcp_s5)*(u(5)-u(6))
  d(T_s6)/dt : Fcn  Expr=(1/tau_s6)*(u(6)-u(7))+(hA_s6/mcp_s6)*(u(5)-u(6))
  d(T_t3)/dt : Fcn  Expr=(2*hA_pb1/mcp_t3)*(u(3)-u(5))-2*hA_s5/mcp_t3*(u(5)-u(6))
  Coolant Exit Temp : Outport
  Fertile Exit Temp : Outport  Port=2
  wires:
  d(T_pb1)/dt/1 -> T_pb1/1
  d(T_pb2)/dt/1 -> T_pb2/1
  d(T_t3)/dt/1 -> T_t3/1
  d(T_s5)/dt/1 -> "T_s5 "/1
  d(T_s6)/dt/1 -> T_s6/1
  T_s6/1 -> Mux/7, Coolant Exit Temp/1
  "T_s5 "/1 -> Mux/6
  T_t3/1 -> Mux/5
  T_pb2/1 -> Fertile Exit Temp/1, Mux/4
  T_pb1/1 -> Mux/3
  Mux/1 -> d(T_s6)/dt/1, d(T_s5)/dt/1, d(T_t3)/dt/1, d(T_pb2)/dt/1, d(T_pb1)/dt/1, To Workspace/1
  Coolant Inlet Temp/1 -> Mux/1
  Fertile Inlet Temp/1 -> Mux/2

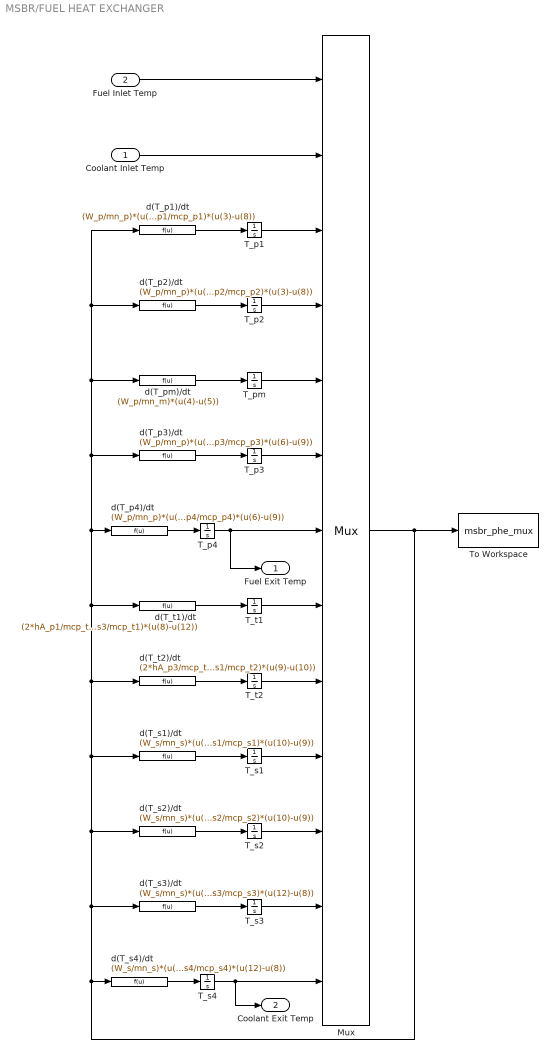
== system MSBR/FUEL HEAT EXCHANGER ==
  Coolant Inlet Temp : Inport
  Fuel Inlet Temp : Inport  Port=2
  Mux : Mux  Inputs=13
      settings: DisplayOption=signals
  T_p1 : Integrator  InitialCondition=T0_p1
  T_p2 : Integrator  InitialCondition=T0_p2
  "T_p3 " : Integrator  InitialCondition=T0_p3
  T_p4 : Integrator  InitialCondition=T0_p4
  T_pm : Integrator  InitialCondition=T0_pm
  T_s1 : Integrator  InitialCondition=T0_s1
  T_s2 : Integrator  InitialCondition=T0_s2
  T_s3 : Integrator  InitialCondition=T0_s3
  T_s4 : Integrator  InitialCondition=T0_s4
  T_t1 : Integrator  InitialCondition=T0_t1
  T_t2 : Integrator  InitialCondition=T0_t2
  To Workspace : ToWorkspace  VariableName=msbr_phe_mux  SampleTime=-1
  d(T_p1)/dt : Fcn  Expr=(W_p/mn_p)*(u(1)-u(3))-(hA_p1/mcp_p1)*(u(3)-u(8))
  d(T_p2)/dt : Fcn  Expr=(W_p/mn_p)*(u(3)-u(4))-(hA_p2/mcp_p2)*(u(3)-u(8))
  d(T_p3)/dt : Fcn  Expr=(W_p/mn_p)*(u(5)-u(6))-(hA_p3/mcp_p3)*(u(6)-u(9))
  d(T_p4)/dt : Fcn  Expr=(W_p/mn_p)*(u(6)-u(7))-(hA_p4/mcp_p4)*(u(6)-u(9))
  d(T_pm)/dt : Fcn  Expr=(W_p/mn_m)*(u(4)-u(5))
  d(T_s1)/dt : Fcn  Expr=(W_s/mn_s)*(u(2)-u(10))-(hA_s1/mcp_s1)*(u(10)-u(9))
  d(T_s2)/dt : Fcn  Expr=(W_s/mn_s)*(u(10)-u(11))-(hA_s2/mcp_s2)*(u(10)-u(9))
  d(T_s3)/dt : Fcn  Expr=(W_s/mn_s)*(u(11)-u(12))-(hA_s3/mcp_s3)*(u(12)-u(8))
  d(T_s4)/dt : Fcn  Expr=(W_s/mn_s)*(u(12)-u(13))-(hA_s4/mcp_s4)*(u(12)-u(8))
  d(T_t1)/dt : Fcn  Expr=(2*hA_p1/mcp_t1)*(u(3)-u(8))-(2*hA_s3/mcp_t1)*(u(8)-u(12))
  d(T_t2)/dt : Fcn  Expr=(2*hA_p3/mcp_t2)*(u(6)-u(9))-(2*hA_s1/mcp_t2)*(u(9)-u(10))
  Fuel Exit Temp : Outport
  Coolant Exit Temp : Outport  Port=2
  wires:
  Fuel Inlet Temp/1 -> Mux/1
  Coolant Inlet Temp/1 -> Mux/2
  d(T_p1)/dt/1 -> T_p1/1
  d(T_p2)/dt/1 -> T_p2/1
  d(T_pm)/dt/1 -> T_pm/1
  d(T_p3)/dt/1 -> "T_p3 "/1
  d(T_p4)/dt/1 -> T_p4/1
  d(T_t1)/dt/1 -> T_t1/1
  d(T_t2)/dt/1 -> T_t2/1
  d(T_s1)/dt/1 -> T_s1/1
  d(T_s2)/dt/1 -> T_s2/1
  T_s2/1 -> Mux/11
  T_s1/1 -> Mux/10
  T_t2/1 -> Mux/9
  T_t1/1 -> Mux/8
  T_p4/1 -> Mux/7, Fuel Exit Temp/1
  "T_p3 "/1 -> Mux/6
  T_pm/1 -> Mux/5
  T_p2/1 -> Mux/4
  T_p1/1 -> Mux/3
  d(T_s3)/dt/1 -> T_s3/1
  d(T_s4)/dt/1 -> T_s4/1
  T_s4/1 -> Coolant Exit Temp/1, Mux/13
  T_s3/1 -> Mux/12
  Mux/1 -> d(T_s4)/dt/1, d(T_s3)/dt/1, d(T_s2)/dt/1, d(T_s1)/dt/1, d(T_t2)/dt/1, d(T_t1)/dt/1, d(T_p4)/dt/1, d(T_p3)/dt/1, d(T_pm)/dt/1, d(T_p2)/dt/1, d(T_p1)/dt/1, To Workspace/1

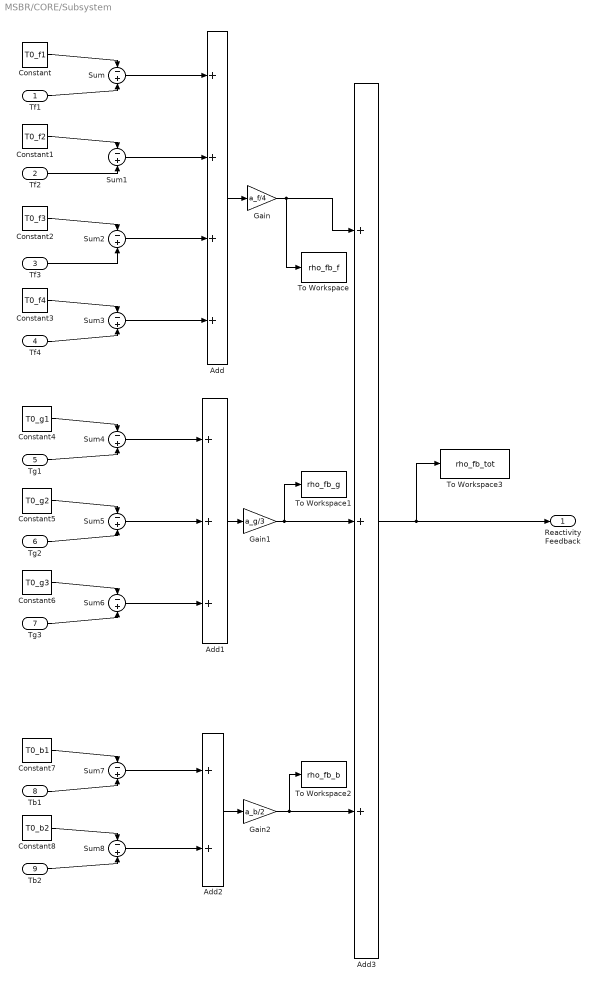
== system MSBR/CORE/Subsystem ==
  Tf1 : Inport
  Tf2 : Inport  Port=2
  Tf3 : Inport  Port=3
  Tf4 : Inport  Port=4
  Tg1 : Inport  Port=5
  Tg2 : Inport  Port=6
  Tg3 : Inport  Port=7
  Tb1 : Inport  Port=8
  Tb2 : Inport  Port=9
  Add : Sum  Inputs=++++
  Add1 : Sum  Inputs=+++
  Add2 : Sum
  Add3 : Sum  Inputs=+++
  Constant : Constant  Value=T0_f1
  Constant1 : Constant  Value=T0_f2
  Constant2 : Constant  Value=T0_f3
  Constant3 : Constant  Value=T0_f4
  Constant4 : Constant  Value=T0_g1
  Constant5 : Constant  Value=T0_g2
  Constant6 : Constant  Value=T0_g3
  Constant7 : Constant  Value=T0_b1
  Constant8 : Constant  Value=T0_b2
  Gain : Gain  Gain=a_f/4
  Gain1 : Gain  Gain=a_g/3
  Gain2 : Gain  Gain=a_b/2
  Sum{,1..8} (9 alike) : Sum  Inputs=-|+
  To Workspace : ToWorkspace  VariableName=rho_fb_f  SampleTime=-1
  To Workspace1 : ToWorkspace  VariableName=rho_fb_g  SampleTime=-1
  To Workspace2 : ToWorkspace  VariableName=rho_fb_b  SampleTime=-1
  To Workspace3 : ToWorkspace  VariableName=rho_fb_tot  SampleTime=-1
  Reactivity Feedback : Outport
  wires:
  Tf1/1 -> Sum/2
  Constant/1 -> Sum/1
  Tf2/1 -> Sum1/2
  Constant1/1 -> Sum1/1
  Tf3/1 -> Sum2/2
  Constant2/1 -> Sum2/1
  Tf4/1 -> Sum3/2
  Constant3/1 -> Sum3/1
  Tg1/1 -> Sum4/2
  Constant4/1 -> Sum4/1
  Tg2/1 -> Sum5/2
  Constant5/1 -> Sum5/1
  Tg3/1 -> Sum6/2
  Constant6/1 -> Sum6/1
  Tb1/1 -> Sum7/2
  Constant7/1 -> Sum7/1
  Tb2/1 -> Sum8/2
  Constant8/1 -> Sum8/1
  Sum/1 -> Add/1
  Sum1/1 -> Add/2
  Sum2/1 -> Add/3
  Sum3/1 -> Add/4
  Sum4/1 -> Add1/1
  Sum5/1 -> Add1/2
  Sum6/1 -> Add1/3
  Sum7/1 -> Add2/1
  Sum8/1 -> Add2/2
  Add/1 -> Gain/1
  Add1/1 -> Gain1/1
  Add2/1 -> Gain2/1
  Gain1/1 -> To Workspace1/1, Add3/2
  Gain/1 -> To Workspace/1, Add3/1
  Gain2/1 -> To Workspace2/1, Add3/3
  Add3/1 -> Reactivity Feedback/1, To Workspace3/1
